simulink model "MyTransmCU_RTW"  (Simulink 9.3)
settings: Solver=ode1  StartTime=0.0  StopTime=inf  FixedStep=0.0002  RelTol=1e-3
PreLoadFcn:
  | vehicle = 'Car'; if ~length(which('cmcmd')), cmenv; end
  | MyTransmCU_RTW_bus
InitFcn:
  | vehicle = 'Car'; if ~length(which('cmcmd')), cmenv; end
  | MyTransmCU_RTW_bus
libraries: simulink x2, CarMaker4SL x1
Description:
  | CarMaker Plug-in Model Target
settings Model: Creator=ml  LastModifiedBy=IPG
settings DataIOCC: LimitDataPoints=on
settings OptimizationCC: ExpressionDepthLimit=2147483647
settings DebuggingCC: StateNameClashWarn=warning  SFExecutionAtInitializationDiag=warning
settings HardwareCC: TargetHWDeviceType=32-bit Generic  ProdEqTarget=off
settings RTWCC: SystemTargetFile=CarMaker.tlc  TemplateMakefile=CarMaker_unix-win64.tmf  Description=CarMaker Plug-in Model Target
settings CodeAppCC: MaxIdLength=127
settings STFCustomTargetCC: GeneratePreprocessorConditionals=Disable all  MultiInstanceERTCode=on  CodeInterfacePackaging=Reusable function  CPPClassGenCompliant=on  GRTInterface=off  GenerateAllocFcn=on  SystemTargetFile=CarMaker.tlc
settings GRTTargetCC: ParMdlRefBuildCompliant=off  CompOptLevelCompliant=off  ConcurrentExecutionCompliant=off  GeneratePreprocessorConditionals=Disable all  MatFileLogging=off  MultiInstanceERTCode=on  CodeInterfacePackaging=Reusable function  GRTInterface=off  GenerateAllocFcn=on  UseToolchainInfoCompliant=off
settings CustomProperty: DataType=string
settings EnumStrPairs: String=Car

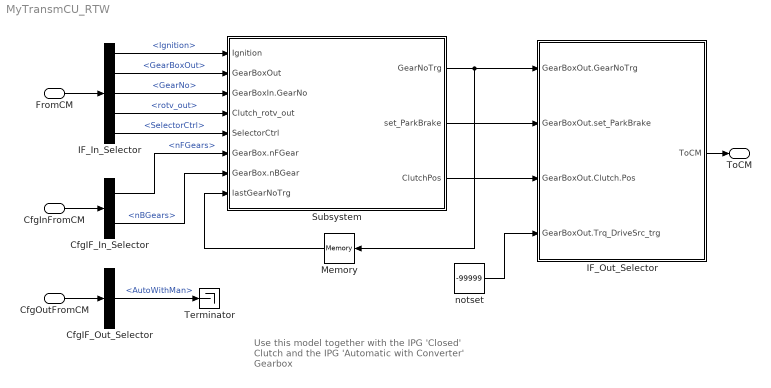
== system MyTransmCU_RTW ==
  note: Use this model together with
      | the IPG 'Closed' Clutch
      | and the IPG 'Automatic with Converter' Gearbox
  FromCM : Inport  OutDataTypeStr=Bus: cmPTTransmCUIn
  CfgInFromCM : Inport  Port=2  OutDataTypeStr=Bus: cmPTTransmCUCfgIn
  CfgOutFromCM : Inport  Port=3  OutDataTypeStr=Bus: cmPTTransmCUCfgOut
  CfgIF_In_Selector : BusSelector  OutputSignals=GearBox.nFGears,GearBox.nBGears
  CfgIF_Out_Selector : BusSelector  OutputSignals=AutoWithMan
  IF_In_Selector : BusSelector  OutputSignals=Ignition,GearBoxOut,GearBoxIn.GearNo,GearBoxIn.Clutch.rotv_out,SelectorCtrl
  IF_Out_Selector : Subsystem  mask(Signal Selection){}
      mask help: Signal Selection Block
      settings: OpenFcn=cmSignalSelect('SignalSelection_CB',gcb)
  Memory : Memory
  Subsystem : Subsystem
  Terminator : Terminator
  notset : Constant  Value=-99999
  ToCM : Outport  OutDataTypeStr=Bus: cmPTTransmCUOut
  wires:
  FromCM/1 -> IF_In_Selector/1
  IF_Out_Selector/1(ToCM) -> ToCM/1
  CfgInFromCM/1 -> CfgIF_In_Selector/1
  CfgOutFromCM/1 -> CfgIF_Out_Selector/1
  CfgIF_Out_Selector/1 -> Terminator/1  "<AutoWithMan>"
  IF_In_Selector/1 -> Subsystem/1(Ignition)  "<Ignition>"
  IF_In_Selector/2 -> Subsystem/2(GearBoxOut)  "<GearBoxOut>"
  IF_In_Selector/3 -> Subsystem/3(GearBoxIn.GearNo)  "<GearNo>"
  Subsystem/1(GearNoTrg) -> Memory/1, IF_Out_Selector/1(GearBoxOut.GearNoTrg)
  Subsystem/2(set_ParkBrake) -> IF_Out_Selector/2(GearBoxOut.set_ParkBrake)
  Subsystem/3(ClutchPos) -> IF_Out_Selector/3(GearBoxOut.Clutch.Pos)
  CfgIF_In_Selector/1 -> Subsystem/6(GearBox.nFGear)  "<nFGears>"
  CfgIF_In_Selector/2 -> Subsystem/7(GearBox.nBGear)  "<nBGears>"
  IF_In_Selector/4 -> Subsystem/4(Clutch_rotv_out)  "<rotv_out>"
  IF_In_Selector/5 -> Subsystem/5(SelectorCtrl)  "<SelectorCtrl>"
  Memory/1 -> Subsystem/8(lastGearNoTrg)
  notset/1 -> IF_Out_Selector/4(GearBoxOut.Trq_DriveSrc_trg)

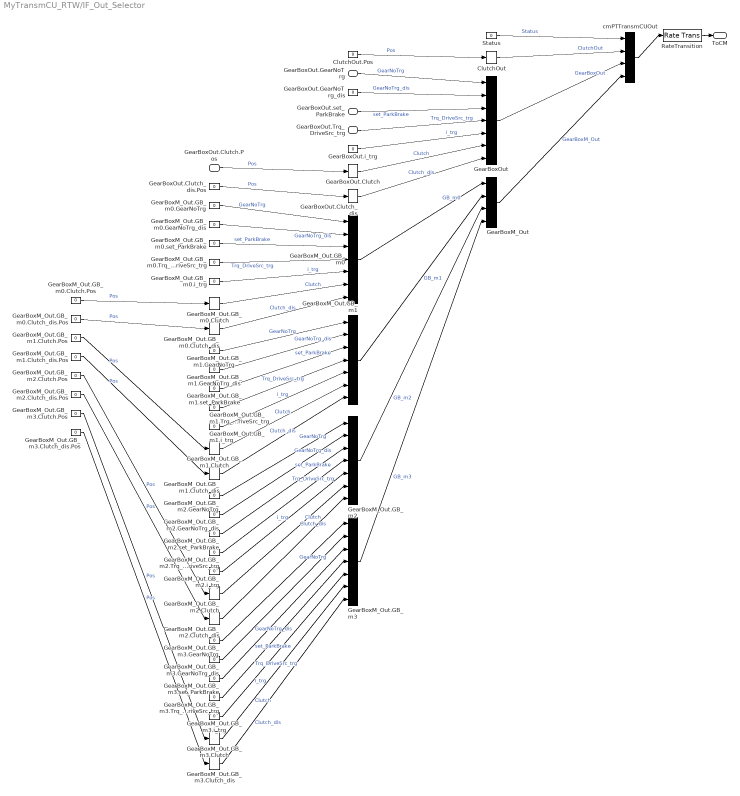
== system MyTransmCU_RTW/IF_Out_Selector ==
  GearBoxOut.GearNoTrg : Inport
  GearBoxOut.set_ParkBrake : Inport  Port=2
  GearBoxOut.Clutch.Pos : Inport  Port=3
  GearBoxOut.Trq_DriveSrc_trg : Inport  Port=4
  ClutchOut : BusCreator  Inputs=1
  ClutchOut.Pos : Constant  Value=0
  GearBoxM_Out : BusCreator  Inputs=4
  GearBoxM_Out.GB_m{0..3} (4 alike) : BusCreator  Inputs=7
  GearBoxM_Out.GB_m0.Clutch : BusCreator  Inputs=1
  GearBoxM_Out.GB_m0.Clutch.Pos : Constant  Value=0
  GearBoxM_Out.GB_m0.Clutch_dis : BusCreator  Inputs=1
  GearBoxM_Out.GB_m0.Clutch_dis.Pos : Constant  Value=0
  GearBoxM_Out.GB_m0.GearNoTrg : Constant  Value=0
  GearBoxM_Out.GB_m0.GearNoTrg_dis : Constant  Value=0
  GearBoxM_Out.GB_m0.Trq_DriveSrc_trg : Constant  Value=0
  GearBoxM_Out.GB_m0.i_trg : Constant  Value=0
  GearBoxM_Out.GB_m0.set_ParkBrake : Constant  Value=0
  GearBoxM_Out.GB_m1.Clutch : BusCreator  Inputs=1
  GearBoxM_Out.GB_m1.Clutch.Pos : Constant  Value=0
  GearBoxM_Out.GB_m1.Clutch_dis : BusCreator  Inputs=1
  GearBoxM_Out.GB_m1.Clutch_dis.Pos : Constant  Value=0
  GearBoxM_Out.GB_m1.GearNoTrg : Constant  Value=0
  GearBoxM_Out.GB_m1.GearNoTrg_dis : Constant  Value=0
  GearBoxM_Out.GB_m1.Trq_DriveSrc_trg : Constant  Value=0
  GearBoxM_Out.GB_m1.i_trg : Constant  Value=0
  GearBoxM_Out.GB_m1.set_ParkBrake : Constant  Value=0
  GearBoxM_Out.GB_m2.Clutch : BusCreator  Inputs=1
  GearBoxM_Out.GB_m2.Clutch.Pos : Constant  Value=0
  GearBoxM_Out.GB_m2.Clutch_dis : BusCreator  Inputs=1
  GearBoxM_Out.GB_m2.Clutch_dis.Pos : Constant  Value=0
  GearBoxM_Out.GB_m2.GearNoTrg : Constant  Value=0
  GearBoxM_Out.GB_m2.GearNoTrg_dis : Constant  Value=0
  GearBoxM_Out.GB_m2.Trq_DriveSrc_trg : Constant  Value=0
  GearBoxM_Out.GB_m2.i_trg : Constant  Value=0
  GearBoxM_Out.GB_m2.set_ParkBrake : Constant  Value=0
  GearBoxM_Out.GB_m3.Clutch : BusCreator  Inputs=1
  GearBoxM_Out.GB_m3.Clutch.Pos : Constant  Value=0
  GearBoxM_Out.GB_m3.Clutch_dis : BusCreator  Inputs=1
  GearBoxM_Out.GB_m3.Clutch_dis.Pos : Constant  Value=0
  GearBoxM_Out.GB_m3.GearNoTrg : Constant  Value=0
  GearBoxM_Out.GB_m3.GearNoTrg_dis : Constant  Value=0
  GearBoxM_Out.GB_m3.Trq_DriveSrc_trg : Constant  Value=0
  GearBoxM_Out.GB_m3.i_trg : Constant  Value=0
  GearBoxM_Out.GB_m3.set_ParkBrake : Constant  Value=0
  GearBoxOut : BusCreator  Inputs=7
  GearBoxOut.Clutch : BusCreator  Inputs=1
  GearBoxOut.Clutch_dis : BusCreator  Inputs=1
  GearBoxOut.Clutch_dis.Pos : Constant  Value=0
  GearBoxOut.GearNoTrg_dis : Constant  Value=0
  GearBoxOut.i_trg : Constant  Value=0
  RateTransition : RateTransition  OutPortSampleTime=str2num(get_param(bdroot,'FixedStep'))
  Status : Constant  Value=0
  cmPTTransmCUOut : BusCreator  Inputs=4
  ToCM : Outport
  wires:
  RateTransition/1 -> ToCM/1
  cmPTTransmCUOut/1 -> RateTransition/1
  Status/1 -> cmPTTransmCUOut/1  "Status"
  ClutchOut/1 -> cmPTTransmCUOut/2  "ClutchOut"
  ClutchOut.Pos/1 -> ClutchOut/1  "Pos"
  GearBoxOut/1 -> cmPTTransmCUOut/3  "GearBoxOut"
  GearBoxOut.GearNoTrg_dis/1 -> GearBoxOut/2  "GearNoTrg_dis"
  GearBoxOut.i_trg/1 -> GearBoxOut/5  "i_trg"
  GearBoxOut.Clutch/1 -> GearBoxOut/6  "Clutch"
  GearBoxOut.Clutch_dis/1 -> GearBoxOut/7  "Clutch_dis"
  GearBoxOut.Clutch_dis.Pos/1 -> GearBoxOut.Clutch_dis/1  "Pos"
  GearBoxM_Out/1 -> cmPTTransmCUOut/4  "GearBoxM_Out"
  GearBoxM_Out.GB_m0/1 -> GearBoxM_Out/1  "GB_m0"
  GearBoxM_Out.GB_m0.GearNoTrg/1 -> GearBoxM_Out.GB_m0/1  "GearNoTrg"
  GearBoxM_Out.GB_m0.GearNoTrg_dis/1 -> GearBoxM_Out.GB_m0/2  "GearNoTrg_dis"
  GearBoxM_Out.GB_m0.set_ParkBrake/1 -> GearBoxM_Out.GB_m0/3  "set_ParkBrake"
  GearBoxM_Out.GB_m0.Trq_DriveSrc_trg/1 -> GearBoxM_Out.GB_m0/4  "Trq_DriveSrc_trg"
  GearBoxM_Out.GB_m0.i_trg/1 -> GearBoxM_Out.GB_m0/5  "i_trg"
  GearBoxM_Out.GB_m0.Clutch/1 -> GearBoxM_Out.GB_m0/6  "Clutch"
  GearBoxM_Out.GB_m0.Clutch.Pos/1 -> GearBoxM_Out.GB_m0.Clutch/1  "Pos"
  GearBoxM_Out.GB_m0.Clutch_dis/1 -> GearBoxM_Out.GB_m0/7  "Clutch_dis"
  GearBoxM_Out.GB_m0.Clutch_dis.Pos/1 -> GearBoxM_Out.GB_m0.Clutch_dis/1  "Pos"
  GearBoxM_Out.GB_m1/1 -> GearBoxM_Out/2  "GB_m1"
  GearBoxM_Out.GB_m1.GearNoTrg/1 -> GearBoxM_Out.GB_m1/1  "GearNoTrg"
  GearBoxM_Out.GB_m1.GearNoTrg_dis/1 -> GearBoxM_Out.GB_m1/2  "GearNoTrg_dis"
  GearBoxM_Out.GB_m1.set_ParkBrake/1 -> GearBoxM_Out.GB_m1/3  "set_ParkBrake"
  GearBoxM_Out.GB_m1.Trq_DriveSrc_trg/1 -> GearBoxM_Out.GB_m1/4  "Trq_DriveSrc_trg"
  GearBoxM_Out.GB_m1.i_trg/1 -> GearBoxM_Out.GB_m1/5  "i_trg"
  GearBoxM_Out.GB_m1.Clutch/1 -> GearBoxM_Out.GB_m1/6  "Clutch"
  GearBoxM_Out.GB_m1.Clutch.Pos/1 -> GearBoxM_Out.GB_m1.Clutch/1  "Pos"
  GearBoxM_Out.GB_m1.Clutch_dis/1 -> GearBoxM_Out.GB_m1/7  "Clutch_dis"
  GearBoxM_Out.GB_m1.Clutch_dis.Pos/1 -> GearBoxM_Out.GB_m1.Clutch_dis/1  "Pos"
  GearBoxM_Out.GB_m2/1 -> GearBoxM_Out/3  "GB_m2"
  GearBoxM_Out.GB_m2.GearNoTrg/1 -> GearBoxM_Out.GB_m2/1  "GearNoTrg"
  GearBoxM_Out.GB_m2.GearNoTrg_dis/1 -> GearBoxM_Out.GB_m2/2  "GearNoTrg_dis"
  GearBoxM_Out.GB_m2.set_ParkBrake/1 -> GearBoxM_Out.GB_m2/3  "set_ParkBrake"
  GearBoxM_Out.GB_m2.Trq_DriveSrc_trg/1 -> GearBoxM_Out.GB_m2/4  "Trq_DriveSrc_trg"
  GearBoxM_Out.GB_m2.i_trg/1 -> GearBoxM_Out.GB_m2/5  "i_trg"
  GearBoxM_Out.GB_m2.Clutch/1 -> GearBoxM_Out.GB_m2/6  "Clutch"
  GearBoxM_Out.GB_m2.Clutch.Pos/1 -> GearBoxM_Out.GB_m2.Clutch/1  "Pos"
  GearBoxM_Out.GB_m2.Clutch_dis/1 -> GearBoxM_Out.GB_m2/7  "Clutch_dis"
  GearBoxM_Out.GB_m2.Clutch_dis.Pos/1 -> GearBoxM_Out.GB_m2.Clutch_dis/1  "Pos"
  GearBoxM_Out.GB_m3/1 -> GearBoxM_Out/4  "GB_m3"
  GearBoxM_Out.GB_m3.GearNoTrg/1 -> GearBoxM_Out.GB_m3/1  "GearNoTrg"
  GearBoxM_Out.GB_m3.GearNoTrg_dis/1 -> GearBoxM_Out.GB_m3/2  "GearNoTrg_dis"
  GearBoxM_Out.GB_m3.set_ParkBrake/1 -> GearBoxM_Out.GB_m3/3  "set_ParkBrake"
  GearBoxM_Out.GB_m3.Trq_DriveSrc_trg/1 -> GearBoxM_Out.GB_m3/4  "Trq_DriveSrc_trg"
  GearBoxM_Out.GB_m3.i_trg/1 -> GearBoxM_Out.GB_m3/5  "i_trg"
  GearBoxM_Out.GB_m3.Clutch/1 -> GearBoxM_Out.GB_m3/6  "Clutch"
  GearBoxM_Out.GB_m3.Clutch.Pos/1 -> GearBoxM_Out.GB_m3.Clutch/1  "Pos"
  GearBoxM_Out.GB_m3.Clutch_dis/1 -> GearBoxM_Out.GB_m3/7  "Clutch_dis"
  GearBoxM_Out.GB_m3.Clutch_dis.Pos/1 -> GearBoxM_Out.GB_m3.Clutch_dis/1  "Pos"
  GearBoxOut.GearNoTrg/1 -> GearBoxOut/1  "GearNoTrg"
  GearBoxOut.set_ParkBrake/1 -> GearBoxOut/3  "set_ParkBrake"
  GearBoxOut.Clutch.Pos/1 -> GearBoxOut.Clutch/1  "Pos"
  GearBoxOut.Trq_DriveSrc_trg/1 -> GearBoxOut/4  "Trq_DriveSrc_trg"

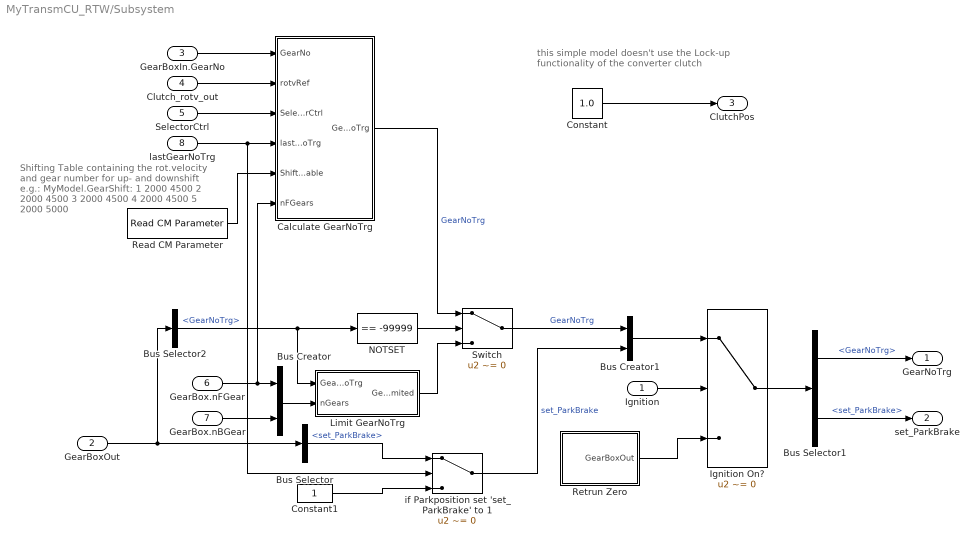
== system MyTransmCU_RTW/Subsystem ==
  note: Shifting Table containing the rot.velocity
      | and gear number for up- and downshift
      | e.g.:
      | MyModel.GearShift:
      |     1    2000    4500
      |     2    2000    4500
      |     3    2000    4500
      |     4    2000    4500
      |     5    2000    5000
  note: this simple model doesn't use the
      | Lock-up functionality of the converter clutch
  Ignition : Inport
  GearBoxOut : Inport  Port=2
  GearBoxIn.GearNo : Inport  Port=3
  Clutch_rotv_out : Inport  Port=4
  SelectorCtrl : Inport  Port=5
  GearBox.nFGear : Inport  Port=6
  GearBox.nBGear : Inport  Port=7
  lastGearNoTrg : Inport  Port=8
  Bus Creator : BusCreator  Inputs=2
  Bus Creator1 : BusCreator  Inputs=2
  Bus Selector : BusSelector  OutputSignals=set_ParkBrake
  Bus Selector1 : BusSelector  OutputSignals=GearNoTrg,set_ParkBrake
  Bus Selector2 : BusSelector  OutputSignals=GearNoTrg
  Calculate GearNoTrg : Subsystem  TreatAsAtomicUnit=on
  Constant : Constant  Value=1.0
  Constant1 : Constant
  Ignition On? : Switch  Criteria=u2 ~= 0
  Limit GearNoTrg : Subsystem
  NOTSET : simulink/Logic and Bit Operations/Compare To Constant  relop===  const=-99999  OutDataTypeStr=uint8
  Read CM Parameter : CarMaker4SL/Read CM Parameter  xfile=Vehicle  xkey=MyModel.GearShift  xnout=80  xdefaults=0  xmuxed=on
      settings: SourceProductName=CarMaker4SL
  Retrun Zero : Subsystem  TreatAsAtomicUnit=on
  Switch : Switch  Criteria=u2 ~= 0
  if Parkposition set 'set_ParkBrake' to 1 : Switch  Criteria=u2 ~= 0
  GearNoTrg : Outport
  set_ParkBrake : Outport  Port=2
  ClutchPos : Outport  Port=3
  wires:
  Constant1/1 -> if Parkposition set 'set_ParkBrake' to 1/3
  Bus Selector/1 -> if Parkposition set 'set_ParkBrake' to 1/1  "<set_ParkBrake>"
  if Parkposition set 'set_ParkBrake' to 1/1 -> Bus Creator1/2  "set_ParkBrake"
  lastGearNoTrg/1 -> if Parkposition set 'set_ParkBrake' to 1/2, Calculate GearNoTrg/4(lastGearNoTrg)
  Limit GearNoTrg/1(GearNoTrg_limited) -> Switch/3
  Calculate GearNoTrg/1(GearNoTrg) -> Switch/1  "GearNoTrg"
  Switch/1 -> Bus Creator1/1  "GearNoTrg"
  Bus Creator1/1 -> Ignition On?/1
  Retrun Zero/1(GearBoxOut) -> Ignition On?/3
  Read CM Parameter/1 -> Calculate GearNoTrg/5(ShiftingTable)
  SelectorCtrl/1 -> Calculate GearNoTrg/3(SelectorCtrl)
  Clutch_rotv_out/1 -> Calculate GearNoTrg/2(rotvRef)
  Ignition/1 -> Ignition On?/2
  Bus Creator/1 -> Limit GearNoTrg/2(nGears)
  Bus Selector2/1 -> Limit GearNoTrg/1(GearNoTrg), NOTSET/1  "<GearNoTrg>"
  NOTSET/1 -> Switch/2
  Constant/1 -> ClutchPos/1
  Bus Selector1/2 -> set_ParkBrake/1  "<set_ParkBrake>"
  Bus Selector1/1 -> GearNoTrg/1  "<GearNoTrg>"
  Ignition On?/1 -> Bus Selector1/1
  GearBoxIn.GearNo/1 -> Calculate GearNoTrg/1(GearNo)
  GearBox.nBGear/1 -> Bus Creator/2
  GearBox.nFGear/1 -> Calculate GearNoTrg/6(nFGears), Bus Creator/1
  GearBoxOut/1 -> Bus Selector2/1, Bus Selector/1

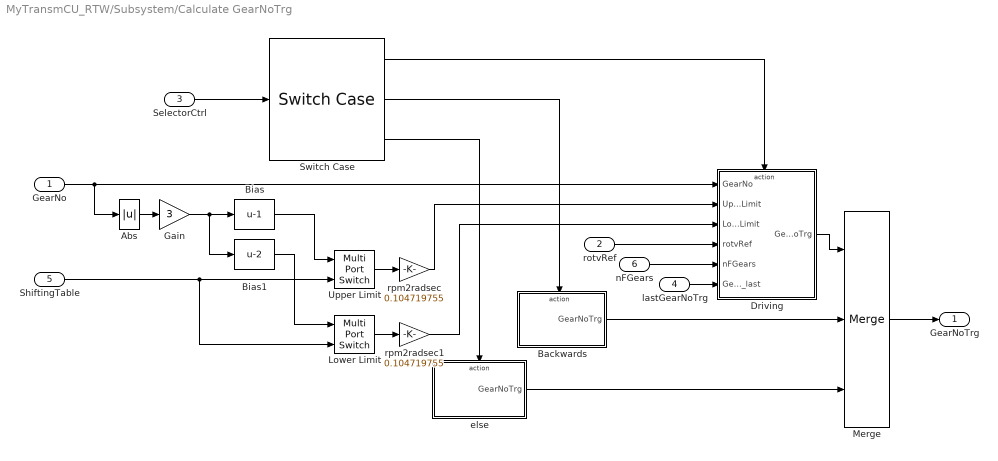
== system MyTransmCU_RTW/Subsystem/Calculate GearNoTrg ==
  GearNo : Inport
  rotvRef : Inport  Port=2
  SelectorCtrl : Inport  Port=3
  lastGearNoTrg : Inport  Port=4
  ShiftingTable : Inport  Port=5
  nFGears : Inport  Port=6
  Abs : Abs
  Backwards : Subsystem  TreatAsAtomicUnit=on
  Bias : Bias  Bias=-1
  Bias1 : Bias  Bias=-2
  Driving : Subsystem  TreatAsAtomicUnit=on
  Gain : Gain  Gain=3
  Lower Limit : MultiPortSwitch  DataPortOrder=Zero-based contiguous  Inputs=1  zeroidx=on
  Merge : Merge  Inputs=3
  Switch Case : SwitchCase  CaseConditions={1,-1}
  Upper Limit : MultiPortSwitch  DataPortOrder=Zero-based contiguous  Inputs=1  zeroidx=on
  else : Subsystem  TreatAsAtomicUnit=on
  rpm2radsec : Gain  Gain=0.104719755
  rpm2radsec1 : Gain  Gain=0.104719755
  GearNoTrg : Outport
  wires:
  lastGearNoTrg/1 -> Driving/6(GearNoTrg_last)
  nFGears/1 -> Driving/5(nFGears)
  rpm2radsec1/1 -> Driving/3(Lower Limit)
  rpm2radsec/1 -> Driving/2(Upper Limit)
  rotvRef/1 -> Driving/4(rotvRef)
  Abs/1 -> Gain/1
  Switch Case/3 -> else/Action
  Switch Case/2 -> Backwards/Action
  Merge/1 -> GearNoTrg/1
  else/1(GearNoTrg) -> Merge/3
  Backwards/1(GearNoTrg) -> Merge/2
  Driving/1(GearNoTrg) -> Merge/1
  Switch Case/1 -> Driving/Action
  SelectorCtrl/1 -> Switch Case/1
  Lower Limit/1 -> rpm2radsec1/1
  GearNo/1 -> Driving/1(GearNo), Abs/1
  Bias1/1 -> Lower Limit/1
  Gain/1 -> Bias1/1, Bias/1
  ShiftingTable/1 -> Lower Limit/2, Upper Limit/2
  Bias/1 -> Upper Limit/1
  Upper Limit/1 -> rpm2radsec/1

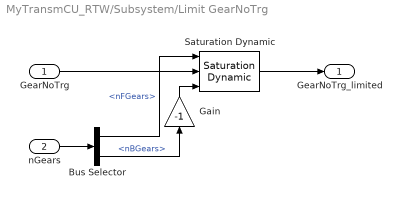
== system MyTransmCU_RTW/Subsystem/Limit GearNoTrg ==
  GearNoTrg : Inport
  nGears : Inport  Port=2
  Bus Selector : BusSelector  OutputSignals=nFGears,nBGears
  Gain : Gain  Gain=-1
  Saturation Dynamic : simulink/Discontinuities/Saturation Dynamic  OutMin=[]  OutMax=[]  OutDataTypeStr=Inherit: Same as second input  OutDataType=sfix(16)  OutScaling=2^-10  DoSatur=off
  GearNoTrg_limited : Outport
  wires:
  nGears/1 -> Bus Selector/1
  Saturation Dynamic/1 -> GearNoTrg_limited/1
  Gain/1 -> Saturation Dynamic/3
  Bus Selector/2 -> Gain/1  "<nBGears>"
  Bus Selector/1 -> Saturation Dynamic/1  "<nFGears>"
  GearNoTrg/1 -> Saturation Dynamic/2

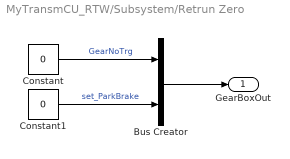
== system MyTransmCU_RTW/Subsystem/Retrun Zero ==
  Bus Creator : BusCreator  Inputs=2
  Constant : Constant  Value=0
  Constant1 : Constant  Value=0
  GearBoxOut : Outport
  wires:
  Bus Creator/1 -> GearBoxOut/1
  Constant1/1 -> Bus Creator/2  "set_ParkBrake"
  Constant/1 -> Bus Creator/1  "GearNoTrg"

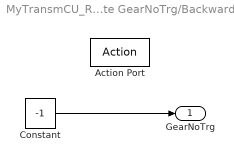
== system MyTransmCU_RTW/Subsystem/Calculate GearNoTrg/Backwards ==
  Action Port : ActionPort  ActionPortLabel=case: { }
  Constant : Constant  Value=-1
  GearNoTrg : Outport  InitialOutput=-1
  wires:
  Constant/1 -> GearNoTrg/1

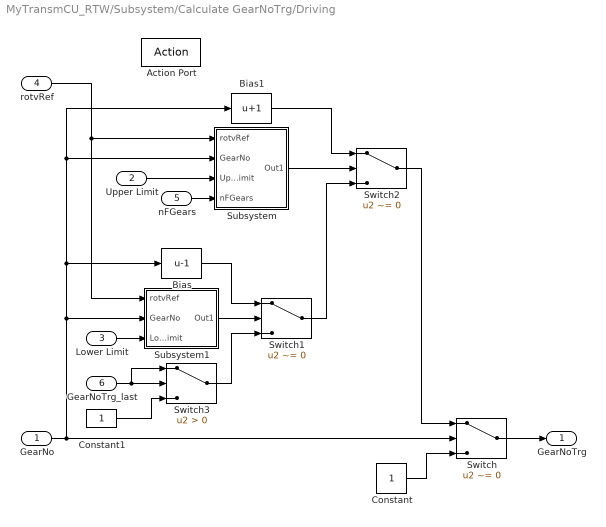
== system MyTransmCU_RTW/Subsystem/Calculate GearNoTrg/Driving ==
  GearNo : Inport
  Upper Limit : Inport  Port=2
  Lower Limit : Inport  Port=3
  rotvRef : Inport  Port=4
  nFGears : Inport  Port=5
  GearNoTrg_last : Inport  Port=6
  Action Port : ActionPort  ActionPortLabel=case: { }
  Bias : Bias  Bias=-1
  Bias1 : Bias  Bias=1
  Constant : Constant
  Constant1 : Constant
  Subsystem : Subsystem
  Subsystem1 : Subsystem
  Switch : Switch  Criteria=u2 ~= 0
  Switch1 : Switch  Criteria=u2 ~= 0
  Switch2 : Switch  Criteria=u2 ~= 0
  Switch3 : Switch  Criteria=u2 > Threshold
  GearNoTrg : Outport
  wires:
  Constant1/1 -> Switch3/3
  GearNoTrg_last/1 -> Switch3/1, Switch3/2
  Switch3/1 -> Switch1/3
  Lower Limit/1 -> Subsystem1/3(Lower Limit)
  Subsystem1/1(Out1) -> Switch1/2
  nFGears/1 -> Subsystem/4(nFGears)
  Upper Limit/1 -> Subsystem/3(Upper Limit)
  Subsystem/1(Out1) -> Switch2/2
  Bias1/1 -> Switch2/1
  Bias/1 -> Switch1/1
  Switch1/1 -> Switch2/3
  Switch2/1 -> Switch/1
  rotvRef/1 -> Subsystem1/1(rotvRef), Subsystem/1(rotvRef)
  Switch/1 -> GearNoTrg/1
  Constant/1 -> Switch/3
  GearNo/1 -> Switch/2, Subsystem1/2(GearNo), Subsystem/2(GearNo), Bias1/1, Bias/1

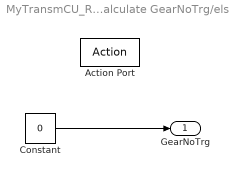
== system MyTransmCU_RTW/Subsystem/Calculate GearNoTrg/else ==
  Action Port : ActionPort  ActionPortLabel=default: { }
  Constant : Constant  Value=0
  GearNoTrg : Outport  InitialOutput=0
  wires:
  Constant/1 -> GearNoTrg/1

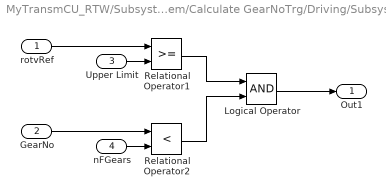
== system MyTransmCU_RTW/Subsystem/Calculate GearNoTrg/Driving/Subsystem ==
  rotvRef : Inport
  GearNo : Inport  Port=2
  Upper Limit : Inport  Port=3
  nFGears : Inport  Port=4
  Logical Operator : Logic  AllPortsSameDT=off  OutDataTypeStr=boolean
  Relational Operator1 : RelationalOperator  OutDataTypeStr=boolean  RndMeth=Nearest
  Relational Operator2 : RelationalOperator  Operator=<  OutDataTypeStr=boolean  RndMeth=Nearest
  Out1 : Outport
  wires:
  Relational Operator2/1 -> Logical Operator/2
  nFGears/1 -> Relational Operator2/2
  GearNo/1 -> Relational Operator2/1
  Logical Operator/1 -> Out1/1
  Relational Operator1/1 -> Logical Operator/1
  Upper Limit/1 -> Relational Operator1/2
  rotvRef/1 -> Relational Operator1/1

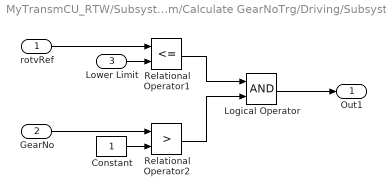
== system MyTransmCU_RTW/Subsystem/Calculate GearNoTrg/Driving/Subsystem1 ==
  rotvRef : Inport
  GearNo : Inport  Port=2
  Lower Limit : Inport  Port=3
  Constant : Constant
  Logical Operator : Logic  AllPortsSameDT=off  OutDataTypeStr=boolean
  Relational Operator1 : RelationalOperator  Operator=<=  OutDataTypeStr=boolean  RndMeth=Nearest
  Relational Operator2 : RelationalOperator  Operator=>  OutDataTypeStr=boolean  RndMeth=Nearest
  Out1 : Outport
  wires:
  Relational Operator2/1 -> Logical Operator/2
  Constant/1 -> Relational Operator2/2
  GearNo/1 -> Relational Operator2/1
  Logical Operator/1 -> Out1/1
  Relational Operator1/1 -> Logical Operator/1
  Lower Limit/1 -> Relational Operator1/2
  rotvRef/1 -> Relational Operator1/1
